simulink model "aeroblock"  (R2016a)
settings: Solver=VariableStepAuto  StartTime=0.0  StopTime=10.0  RelTol=1e-3
libraries: aerolibanim x2, aerolib6dof2 x1, aerolibconvert2 x1
settings Model: Creator=GusBus  LastModifiedBy=GusBus

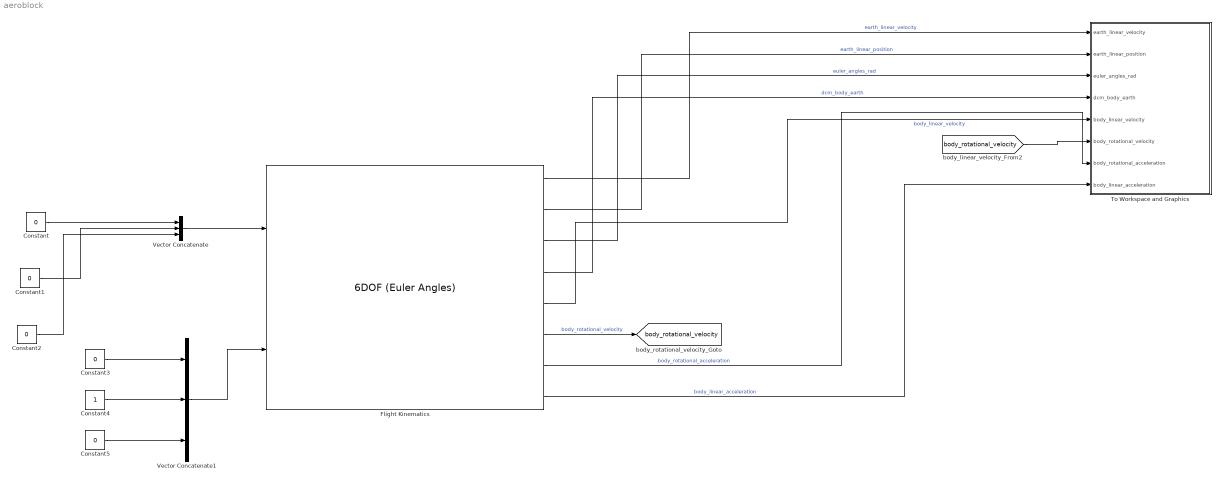
== system aeroblock ==
  Constant{,1..3,5} (5 alike) : Constant  Value=0
  Constant4 : Constant
  Flight Kinematics : aerolib6dof2/6DOF (Euler Angles)  units=Metric (MKS)  mtype=Fixed  rep=Euler Angles  xme_0=[0 0 1]  Vm_0=[0 0 0]  eul_0=[0 0 0]  pm_0=[0 0 0]  mass_0=2.2  mass_e=0.5  mass_f=2.0  inertia=[0.5 0 0; 0 0.5 0; 0 0 0.85]  inertia_e=eye(3)  inertia_f=2*eye(3)  k_quat=1.0  vre_flag=on
  To Workspace and Graphics : Subsystem
  Vector Concatenate : Concatenate  NumInputs=3
  Vector Concatenate1 : Concatenate  NumInputs=3
  tag scope: body_rotational_velocity=global
  wires:
  Constant/1 -> Vector Concatenate/1
  Constant1/1 -> Vector Concatenate/2
  Constant2/1 -> Vector Concatenate/3
  Constant3/1 -> Vector Concatenate1/1
  Constant4/1 -> Vector Concatenate1/2
  Constant5/1 -> Vector Concatenate1/3
  Vector Concatenate1/1 -> Flight Kinematics/2
  Vector Concatenate/1 -> Flight Kinematics/1
  Flight Kinematics/4 -> To Workspace and Graphics/4(dcm_body_earth)  "dcm_body_earth"
  Flight Kinematics/5 -> To Workspace and Graphics/5(body_linear_velocity)  "body_linear_velocity"
  Flight Kinematics/1 -> To Workspace and Graphics/1(earth_linear_velocity)  "earth_linear_velocity"
  Flight Kinematics/2 -> To Workspace and Graphics/2(earth_linear_position)  "earth_linear_position"
  Flight Kinematics/3 -> To Workspace and Graphics/3(euler_angles_rad)  "euler_angles_rad"
  Flight Kinematics/6 -> [body_rotational_velocity]  "body_rotational_velocity"
  Flight Kinematics/7 -> To Workspace and Graphics/7(body_rotational_acceleration)  "body_rotational_acceleration"
  Flight Kinematics/8 -> To Workspace and Graphics/8(body_linear_acceleration)  "body_linear_acceleration"
  [body_rotational_velocity] -> To Workspace and Graphics/6(body_rotational_velocity)

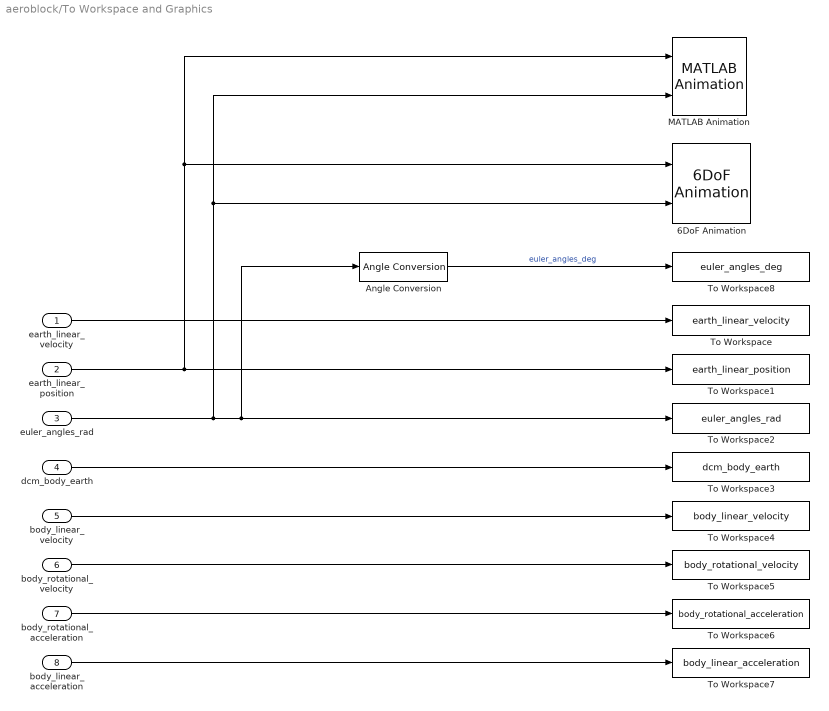
== system aeroblock/To Workspace and Graphics ==
  earth_linear_velocity : Inport
  earth_linear_position : Inport  Port=2
  euler_angles_rad : Inport  Port=3
  dcm_body_earth : Inport  Port=4
  body_linear_velocity : Inport  Port=5
  body_rotational_velocity : Inport  Port=6
  body_rotational_acceleration : Inport  Port=7
  body_linear_acceleration : Inport  Port=8
  6DoF Animation : aerolibanim/6DoF Animation  u1=[0 4000 -2000 2000 -5000 -3000]  u2=0.1  u3=1.0  u4=[4000 0 -5000]  u5=Fixed position  u6=[3000 3000 3000]  u7=90  u8=off
  Angle Conversion : aerolibconvert2/Angle Conversion  IU=rad  OU=deg
  MATLAB Animation : aerolibanim/MATLAB Animation  Tag=Matlab Animation 6 DOF  Vehicles=1  Geometries='astredwedge.mat'  BoundingBoxCoordinates=[-50,50,-50,50,-50,50]  CameraOffset=[-15,-15,0]  CameraViewAngle=135  SampleTime=0.01  FigurePosition=[2,42,958,981]
  To Workspace : ToWorkspace  VariableName=earth_linear_velocity  SampleTime=-1
  To Workspace1 : ToWorkspace  VariableName=earth_linear_position  SampleTime=-1
  To Workspace2 : ToWorkspace  VariableName=euler_angles_rad  SampleTime=-1
  To Workspace3 : ToWorkspace  VariableName=dcm_body_earth  SampleTime=-1
  To Workspace4 : ToWorkspace  VariableName=body_linear_velocity  SampleTime=-1
  To Workspace5 : ToWorkspace  VariableName=body_rotational_velocity  SampleTime=-1
  To Workspace6 : ToWorkspace  VariableName=body_rotational_acceleration  SampleTime=-1
  To Workspace7 : ToWorkspace  VariableName=body_linear_acceleration  SampleTime=-1
  To Workspace8 : ToWorkspace  VariableName=euler_angles_deg  SampleTime=-1
  wires:
  body_linear_velocity/1 -> To Workspace4/1
  dcm_body_earth/1 -> To Workspace3/1
  body_rotational_velocity/1 -> To Workspace5/1
  body_linear_acceleration/1 -> To Workspace7/1
  earth_linear_position/1 -> 6DoF Animation/1, MATLAB Animation/1, To Workspace1/1
  euler_angles_rad/1 -> 6DoF Animation/2, MATLAB Animation/2, To Workspace2/1, Angle Conversion/1
  body_rotational_acceleration/1 -> To Workspace6/1
  earth_linear_velocity/1 -> To Workspace/1
  Angle Conversion/1 -> To Workspace8/1  "euler_angles_deg"
